simulink model "fp_mul"  (Simulink 7.6)
settings: Solver=FixedStepDiscrete  StartTime=0.0  StopTime=1  FixedStep=1  RelTol=1e-3
settings Model: Creator=jordan  LastModifiedBy=jordan
settings DataIOCC: LimitDataPoints=off  SaveOutput=off  SignalLogging=off  DSMLogging=off  SaveTime=off
settings OptimizationCC: BlockReduction=off  ConditionallyExecuteInputs=off

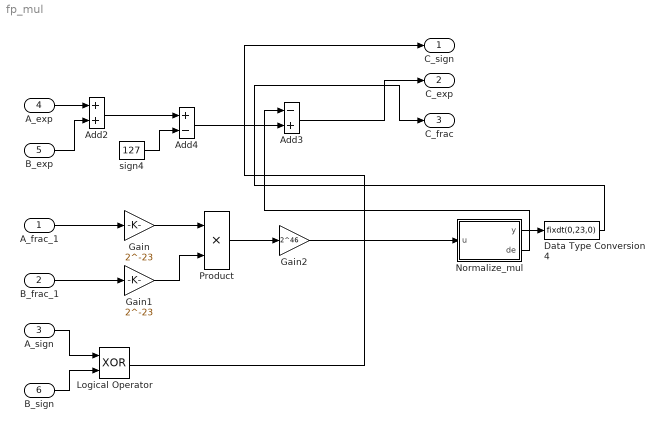
== system fp_mul ==
  A_frac_1 : Inport  OutDataTypeStr=fixdt(0,24,0)
  B_frac_1 : Inport  Port=2  OutDataTypeStr=fixdt(0,24,0)
  A_sign : Inport  Port=3  OutDataTypeStr=boolean
  A_exp : Inport  Port=4  OutDataTypeStr=uint8
  B_exp : Inport  Port=5  OutDataTypeStr=uint8
  B_sign : Inport  Port=6  OutDataTypeStr=boolean
  Add2 : Sum  OutDataTypeStr=fixdt(0,9,0)  RndMeth=Nearest  SaturateOnIntegerOverflow=on
  Add3 : Sum  Inputs=-+  OutDataTypeStr=uint8  RndMeth=Nearest  SaturateOnIntegerOverflow=on
  Add4 : Sum  Inputs=+-  OutDataTypeStr=uint8  RndMeth=Nearest  SaturateOnIntegerOverflow=on
  Data Type Conversion4 : DataTypeConversion  OutDataTypeStr=fixdt(0,23,0)  RndMeth=Nearest
  Gain : Gain  Gain=2^-23  OutDataTypeStr=fixdt(0,24,23)  RndMeth=Nearest
  Gain1 : Gain  Gain=2^-23  OutDataTypeStr=fixdt(0,24,23)  RndMeth=Nearest
  Gain2 : Gain  Gain=2^46  OutDataTypeStr=fixdt(0,48,0)  RndMeth=Nearest  SaturateOnIntegerOverflow=on
  Logical Operator : Logic  Operator=XOR  AllPortsSameDT=off  OutDataTypeStr=boolean
  Normalize_mul : Stateflow chart  TreatAsAtomicUnit=on
  Product : Product  OutDataTypeStr=fixdt(0,48,46)  RndMeth=Nearest  SaturateOnIntegerOverflow=on
  sign4 : Constant  Value=127  OutDataTypeStr=fixdt(0,9,0)
  C_sign : Outport  OutDataTypeStr=boolean
  C_exp : Outport  Port=2  OutDataTypeStr=uint8
  C_frac : Outport  Port=3  OutDataTypeStr=fixdt(0,23,0)
  wires:
  B_exp/1 -> Add2/2
  Normalize_mul/1(y) -> Data Type Conversion4/1
  Normalize_mul/2(de) -> Add3/1
  Add3/1 -> C_exp/1
  Data Type Conversion4/1 -> C_frac/1
  Logical Operator/1 -> C_sign/1
  Product/1 -> Gain2/1
  Add2/1 -> Add4/1
  sign4/1 -> Add4/2
  Add4/1 -> Add3/2
  Gain/1 -> Product/1
  Gain1/1 -> Product/2
  Gain2/1 -> Normalize_mul/1(u)
  A_frac_1/1 -> Gain/1
  B_frac_1/1 -> Gain1/1
  A_sign/1 -> Logical Operator/1
  A_exp/1 -> Add2/1
  B_sign/1 -> Logical Operator/2

== matlab function Normalize_mul ==
  data: u input fixdt(0,48,0); y output uint32; de output double
function [y,de] = fcn(u)
%#eml

buf=u;
p=int8(-1);
c=bitand(buf,fi(2^47,0,48,0));
for ind=1:25
    if (c==0)
        p=p+1;
        buf=bitshift(buf,1);
        c=bitand(buf,fi(2^47,0,48,0));
    end
end
bufy = bitand(bitshift(u,p),fi(2^46-1,0,48,0));
y=uint32(bitshift(bufy,-23));
de=p;
